simulink model "ex19_5"  (R2025a)
settings: Solver=VariableStepAuto  StartTime=0.0  StopTime=3.6e-3  FixedStep=1/(2.5e3)  RelTol=1e-6
undefined symbols (not defined in the file or in its folder): a, K
libraries: spsTriangleGeneratorLib x1
settings Model: Creator=eechris  LastModifiedBy=eechris
settings RTWCC: GPUComputeCapability=3.5

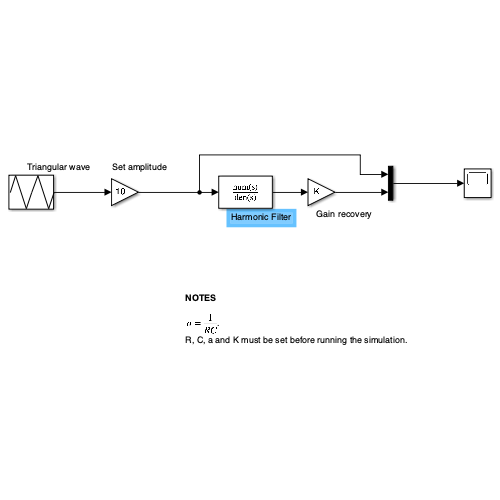
[thumbnail: Simulink's stored preview of the top-level diagram]
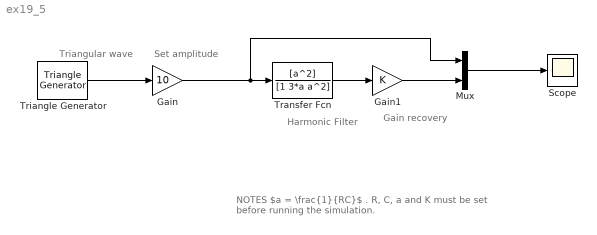
== system ex19_5 ==
  note: Set amplitude
  note: Triangular wave
  note: Gain recovery
  note: Harmonic Filter
  note: NOTES
      |
      | $a = \frac{1}{RC}$ .
      | R, C, a and K must be set before running the simulation.
  Gain : Gain  Gain=10
  Gain1 : Gain  Gain=K
  Mux : Mux  Inputs=2
  Scope : Scope
      settings: ActiveDisplayYMinimum=-13.268606683091498  ActiveDisplayYMaximum=18.078201568437734
  Transfer Fcn : TransferFcn  Numerator=[a^2]  Denominator=[1 3*a a^2]
  Triangle Generator : spsTriangleGeneratorLib/Triangle Generator  Freq=2.5e3  Phase=90  Ts=0
  wires:
  Triangle Generator/1 -> Gain/1
  Gain/1 -> Transfer Fcn/1, Mux/1
  Transfer Fcn/1 -> Gain1/1
  Mux/1 -> Scope/1
  Gain1/1 -> Mux/2
